simulink model "HW3"  (R2020a)
settings: Solver=ode1  StartTime=0.0  StopTime=10.0  RelTol=1e-3  EnableMultiTasking=on
libraries: arduinolib x2, THLlib x1
settings Model: SILPILModeSetting=veronly  ExtModeTrigDuration=2  Creator=da_co  LastModifiedBy=da_co
settings OptimizationCC: EnhancedBackFolding=on  PassReuseOutputArgsAs=Individual arguments  ZeroExternalMemoryAtStartup=off  ZeroInternalMemoryAtStartup=off  MaxStackSize=64  OptimizeBlockOrder=speed  DifferentSizesBufferReuse=on  OptimizationCustomize=off  EfficientTunableParamExpr=on
settings DebuggingCC: ParameterTunabilityLossMsg=error
settings HardwareCC: ProdBitPerInt=16  ProdBitPerPointer=16  ProdBitPerSizeT=16  ProdBitPerPtrDiffT=16  ProdLargestAtomicFloat=None  ProdWordSize=8  ProdHWDeviceType=Atmel->AVR  UseSimulinkCoderFeatures=off
settings SFSimCC: MATLABDynamicMemAlloc=off
settings RTWCC: SystemTargetFile=ert.tlc  HardwareBoard=Arduino Mega 2560  TLCOptions=-aInlineSetEventsForThisBaseRateFcn=TLC_FALSE -aSuppressMultiTaskScheduler=TLC_FALSE -aRateBasedStepFcn=1  TemplateMakefile=ert_default_tmf  Toolchain=Arduino AVR  BuildConfiguration=Faster Runs
settings CodeAppCC: ForceParamTrailComments=on  IgnoreCustomStorageClasses=off  OperatorAnnotations=on  SimulinkDataObjDesc=on  SFDataObjDesc=on  InsertBlockDesc=on
settings ERTTargetCC: SupportContinuousTime=on  SupportVariableSizeSignals=on  ExtModeStaticAllocSize=2048

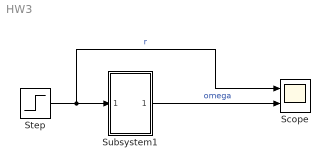
== system HW3 ==
  Scope : Scope  NumInputPorts=2
  Step : Step  After=10  SampleTime=0
  Subsystem1 : Subsystem
  wires:
  Step/1 -> Scope/1, Subsystem1/1(In1)  "r"
  Subsystem1/1(Out1) -> Scope/2  "omega"

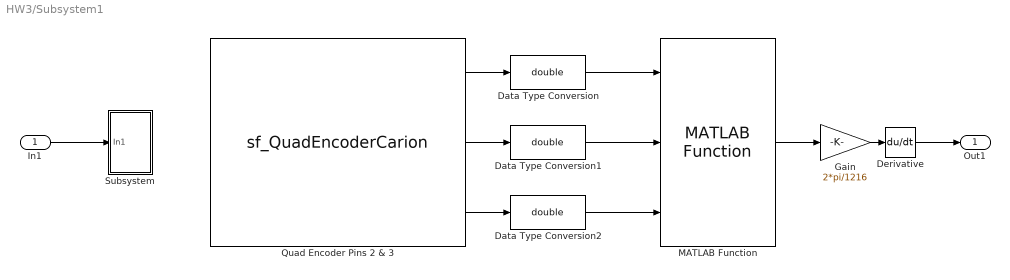
== system HW3/Subsystem1 ==
  In1 : Inport
  Data Type Conversion : DataTypeConversion  OutDataTypeStr=double
  Data Type Conversion1 : DataTypeConversion  OutDataTypeStr=double
  Data Type Conversion2 : DataTypeConversion  OutDataTypeStr=double
  Derivative : Derivative
  Gain : Gain  Gain=2*pi/1216
  MATLAB Function : THLlib/QuadEncoder/MATLAB Function  SystemSampleTime=-1  Latency=0  AutoFrameSizeCalculation=off
      settings: SourceProductName=Take Home Labs Arduino Support Package
  Quad Encoder Pins 2 & 3 : S-Function  InitFcn=try, set_param(gcb,'FunctionName','sf_QuadEncoderCarion'), end  FunctionName=sf_QuadEncoderCarion  Parameters=uint8(0),uint8(2),uint8(3)  SFunctionModules=sf_QuadEncoderCarion_wrapper  SFunctionDeploymentMode=off  EnableBusSupport=off  mask(S-Function Builder){}
      mask init:
      | val = [[.9  0.75 0.75 1 1 .9 .9 1]',[1 1 0.75 0.75 .9 .9 1 .9]'];try , sys = get_param(gcb,'SfunBuilderFcnName');if isempty(sys), sys = get_param(gcb,'FunctionName'); end,catch, sys = get_param(gcb,'FunctionName'); end
      settings: CopyFcn=set_param(gcbh,'LinkStatus','none')  PreSaveFcn=try, set_param(gcb,'FunctionName','sf_QuadEncoderCarion'), end  OpenFcn=sfunctionwizard(gcbh)
      mask Display: plot(val(:,1),val(:,2)),disp(sys), port_label('output',1,'pos'), port_label('output',2,'overflow'), port_label('output',3,'underflow')
  Subsystem : Subsystem
  Out1 : Outport
  wires:
  Data Type Conversion1/1 -> MATLAB Function/2
  MATLAB Function/1 -> Gain/1
  Quad Encoder Pins 2 & 3/1 -> Data Type Conversion/1
  Data Type Conversion2/1 -> MATLAB Function/3
  Derivative/1 -> Out1/1
  Gain/1 -> Derivative/1
  In1/1 -> Subsystem/1(In1)
  Quad Encoder Pins 2 & 3/2 -> Data Type Conversion1/1
  Data Type Conversion/1 -> MATLAB Function/1
  Quad Encoder Pins 2 & 3/3 -> Data Type Conversion2/1

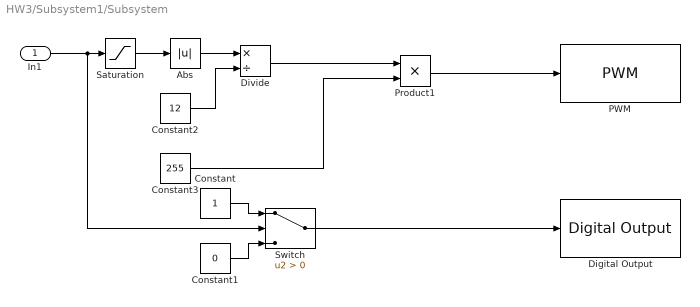
== system HW3/Subsystem1/Subsystem ==
  In1 : Inport
  Abs : Abs
  Constant : Constant
  Constant1 : Constant  Value=0
  Constant2 : Constant  Value=12
  Constant3 : Constant  Value=255
  Digital Output : arduinolib/Digital Output  pinNumber=4  Direction=output  blockPlatform=arduino
  Divide : Product  Inputs=*/
  PWM : arduinolib/PWM  pinNumber=5  frequencyType=Default  desiredFrequency=490.2  achievableFrequency=490.2
  Product1 : Product
  Saturation : Saturate  UpperLimit=12  LowerLimit=-12
  Switch : Switch  Criteria=u2 > Threshold
  wires:
  Switch/1 -> Digital Output/1
  Constant/1 -> Switch/1
  Product1/1 -> PWM/1
  In1/1 -> Saturation/1, Switch/2
  Saturation/1 -> Abs/1
  Divide/1 -> Product1/1
  Constant1/1 -> Switch/3
  Constant3/1 -> Product1/2
  Abs/1 -> Divide/1
  Constant2/1 -> Divide/2
